simulink model "main"  (R2024b)
settings: Solver=VariableStepAuto  StartTime=0.0  StopTime=10.0  RelTol=1e-3
undefined symbols (not defined in the file): matlabshared
libraries: drivingscenarioandsensors x3, autolibshared x1
settings Model: Creator=maciej  LastModifiedBy=maciej

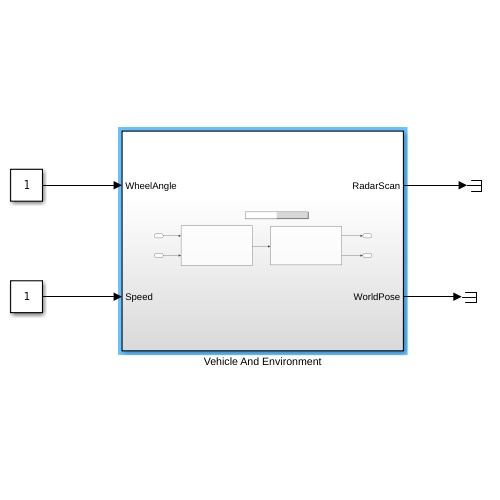
[thumbnail: Simulink's stored preview of the top-level diagram]
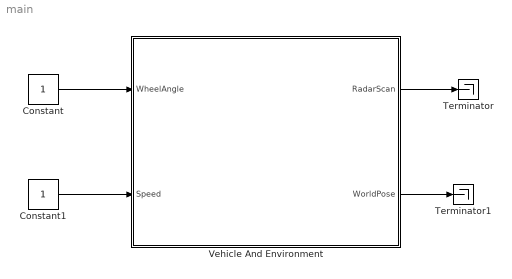
== system main ==
  Constant : Constant
  Constant1 : Constant
  Terminator : Terminator
  Terminator1 : Terminator
  Vehicle And Environment : Subsystem
  wires:
  Constant/1 -> Vehicle And Environment/1(WheelAngle)
  Constant1/1 -> Vehicle And Environment/2(Speed)
  Vehicle And Environment/1(RadarScan) -> Terminator/1
  Vehicle And Environment/2(WorldPose) -> Terminator1/1

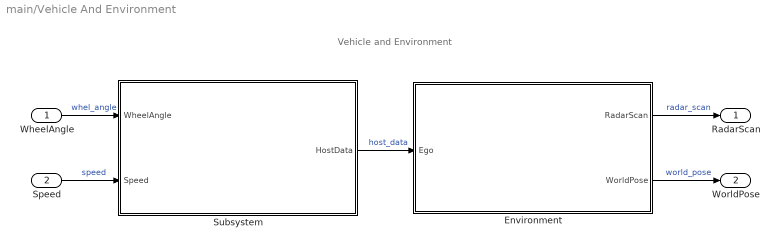
== system main/Vehicle And Environment ==
  note: Vehicle and Environment
  WheelAngle : Inport
  Speed : Inport  Port=2
  Environment : Subsystem
  Subsystem : Subsystem
  RadarScan : Outport
  WorldPose : Outport  Port=2
  wires:
  Environment/2(WorldPose) -> WorldPose/1  "world_pose"
  Environment/1(RadarScan) -> RadarScan/1  "radar_scan"
  Subsystem/1(HostData) -> Environment/1(Ego)  "host_data"
  Speed/1 -> Subsystem/2(Speed)  "speed"
  WheelAngle/1 -> Subsystem/1(WheelAngle)  "whel_angle"

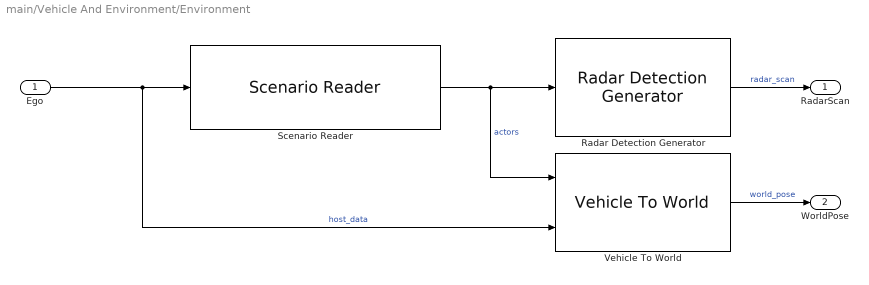
== system main/Vehicle And Environment/Environment ==
  Ego : Inport
  Radar Detection Generator : drivingscenarioandsensors/Radar Detection Generator  SensorIndex=1  UpdateInterval=0.1  SensorLocation=[ 3.4, 0 ]  Height=0.2  Yaw=0  Pitch=0  Roll=0  BusNameSource=Auto  BusName=BusRadarDetectionGenerator  MaxNumDetectionsSource=Property  MaxNumDetections=128  DetectionCoordinates=Ego Cartesian  SimulateUsing=Interpreted execution  AzimuthResolution=4  ElevationResolution=10  RangeResolution=2.5  RangeRateResolution=0.5  AzimuthBiasFraction=0.1  ElevationBiasFraction=0.1  RangeBiasFraction=0.05  RangeRateBiasFraction=0.05  FieldOfView=[ 20, 5 ]  MaxRange=150  RangeRateLimits=[ -100, 100 ]  DetectionProbability=0.9  FalseAlarmRate=1e-6  ReferenceRange=100  ReferenceRCS=0  HasElevation=off  HasRangeRate=on  HasNoise=on  HasFalseAlarms=on  HasOcclusion=on  InitialSeedSource=Repeatable  InitialSeed=0  UsedSeed=matlabshared.tracking.internal.SimulinkUtilities.seedManager(gcb)  ActorProfilesSource=Parameters  ActorProfilesParameters=driving.internal.ActorProfilesRadarParameters  ActorProfilesExpression=struct( 'ClassID', 0, 'Length', 4.7, 'Width', 1.8, 'Height', 1.4, 'OriginOffset', [ -1.35, 0, 0 ], 'RCSPattern', [ 10, 10; 10, 10 ], 'RCSAzimuthAngles', [ -180, 180 ], 'RCSElevationAngles', [ -90, 90 ] )
  Scenario Reader : drivingscenarioandsensors/Scenario Reader  ScenarioSource=From file  ScenarioFileName=/home/maciej/MATLAB/Projects/cbf_parking/scenarios/scenario_1.mat  ScenarioVariableName=scenario  OutputCoordinateSystem=Vehicle coordinates  EgoVehicleSource=Input port  EgoVehicleActorID=1  OrientVehiclesOnRoad=off  OutputEgoVehiclePose=on  OutputEgoVehicleState=off  SampleTime=0.01  LaneBoundaryOutput=None  LaneBoundaryDistance=0:0.5:9.5  LaneBoundaryLocation=Center of lane markings  BusNameSource=Property  BusName=BusActors  BusNumActorsSource=Scenario  BusNumActors=100  BusName2Source=Auto  BusName2=BusLaneBoundaries  BusNumLaneBoundariesSource=Scenario  BusNumLaneBoundaries=10  BusName3Source=Auto  BusName3=BusEgoActor  BusName4Source=Auto  BusName4=BusEgoState  ShowCoordinateLabels=on  SimulateUsing=Interpreted execution
  Vehicle To World : drivingscenarioandsensors/Vehicle To World  BusNameSource=Property  BusName=BusVehicleToWorldActors  SimulateUsing=Interpreted execution
  RadarScan : Outport
  WorldPose : Outport  Port=2
  wires:
  Vehicle To World/1 -> WorldPose/1  "world_pose"
  Scenario Reader/1 -> Radar Detection Generator/1, Vehicle To World/1  "actors"
  Ego/1 -> Scenario Reader/1, Vehicle To World/2  "host_data"
  Radar Detection Generator/1 -> RadarScan/1  "radar_scan"

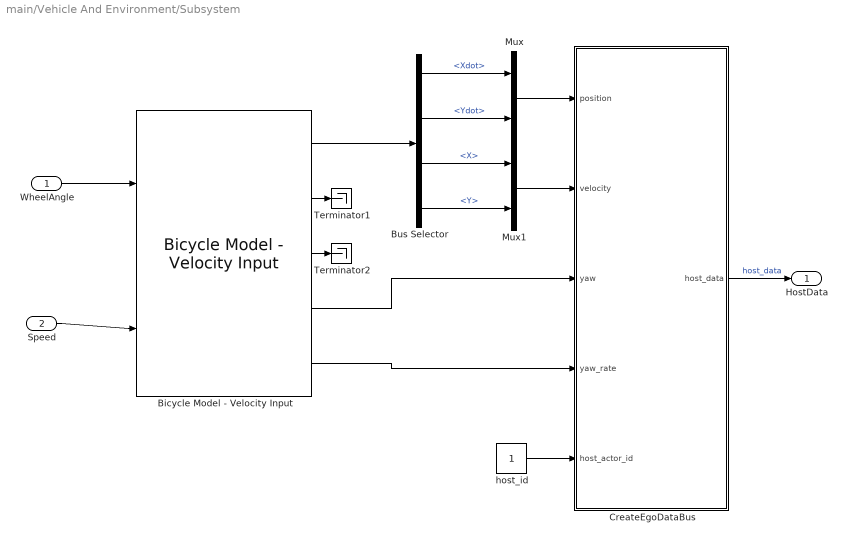
== system main/Vehicle And Environment/Subsystem ==
  WheelAngle : Inport
  Speed : Inport  Port=2
  Bicycle Model - Velocity Input : autolibshared/Bicycle Model - Velocity Input  trackMode=Single (bicycle)  inputMode=External longitudinal velocity  frontSteerMode=on  rearSteerMode=off  windMode=off  muMode=off  extFMode=off  extMMode=off  aMode=3  NF=2  NR=2  m=2000  a=1.4  b=1.6  h=0.35  X_o=0  xdot_o=0  CalphaMode=off  sigmaMode=on  w=[1.4,1.4]  Cy_f=12e3  Cy_r=11e3  sigma_f=.1  sigma_r=.1  alpha_f_brk=[-.1 .1]  Cy_f_data=[-9e3 9e3]  alpha_r_brk=[-.1 .1]  Cy_r_data=[-9e3 9e3]  Y_o=0  ydot_o=0  Izz=4000  psi_o=0  r_o=0  Af=2  Cd=.3  Cl=.1  Cpm=.1  beta_w=[0 0.01:0.01:0.3]  Cs=[0 0.01:0.01:0.3]  Cym=[0 1e-6:0.01:0.3]  Pabs=101325  Tair=273  g=9.81  mu=1  xdot_tol=.01  Fznom=5000  Fxtire_sat=1e6  Fytire_sat=1e6  longOff=0  latOff=0  vertOff=0
      settings: LibrarySourceBlock=drivingscenarioandsensors/Bicycle Model - Velocity Input
  Bus Selector : BusSelector  OutputSignals=InertFrm.RearAxl.Vel.Xdot,InertFrm.RearAxl.Vel.Ydot,InertFrm.RearAxl.Disp.X,InertFrm.RearAxl.Disp.Y
  CreateEgoDataBus : MATLAB Function  TreatAsAtomicUnit=on
  Mux : Mux  Inputs=2
  Mux1 : Mux  Inputs=2
  Terminator1 : Terminator
  Terminator2 : Terminator
  host_id : Constant
  HostData : Outport
  wires:
  Bicycle Model - Velocity Input/3 -> Terminator2/1
  Bicycle Model - Velocity Input/1 -> Bus Selector/1
  CreateEgoDataBus/1(host_data) -> HostData/1  "host_data"
  Bicycle Model - Velocity Input/5 -> CreateEgoDataBus/4(yaw_rate)
  Speed/1 -> Bicycle Model - Velocity Input/2
  WheelAngle/1 -> Bicycle Model - Velocity Input/1
  Bicycle Model - Velocity Input/2 -> Terminator1/1
  Bicycle Model - Velocity Input/4 -> CreateEgoDataBus/3(yaw)
  host_id/1 -> CreateEgoDataBus/5(host_actor_id)
  Mux/1 -> CreateEgoDataBus/1(position)
  Bus Selector/1 -> Mux/1  "<Xdot>"
  Bus Selector/2 -> Mux/2  "<Ydot>"
  Mux1/1 -> CreateEgoDataBus/2(velocity)
  Bus Selector/4 -> Mux1/2  "<Y>"
  Bus Selector/3 -> Mux1/1  "<X>"

== matlab function main/Vehicle And Environment/Subsystem/CreateEgoDataBus ==
  data: position input double; host_data output Bus: EgoData; velocity input double; yaw input double; yaw_rate input double; host_actor_id input double
function host_data = CreateEgoDataBus(position, velocity, yaw, yaw_rate, host_actor_id)
% Pack ego information into a single ego actor bus
%
% Imoprtant note:
% Output is a bus of type EgoData. This is the same bus used by the
% Scenario Reader to output an individual actor.

host_data = struct(...
    'ActorID', host_actor_id,...
    'Position', [position(1) position(2) 0], ...
    'Velocity', [velocity(1) velocity(2) 0], ...
    'Roll', 0, ...
    'Pitch', 0, ...
    'Yaw', yaw, ...
    'AngularVelocity', [0 0 yaw_rate]);
